simulink model "schemat_4"  (R2018a)
settings: Solver=VariableStepAuto  StartTime=0.0  StopTime=20  RelTol=1e-3
settings Model: Creator=HP  LastModifiedBy=HP

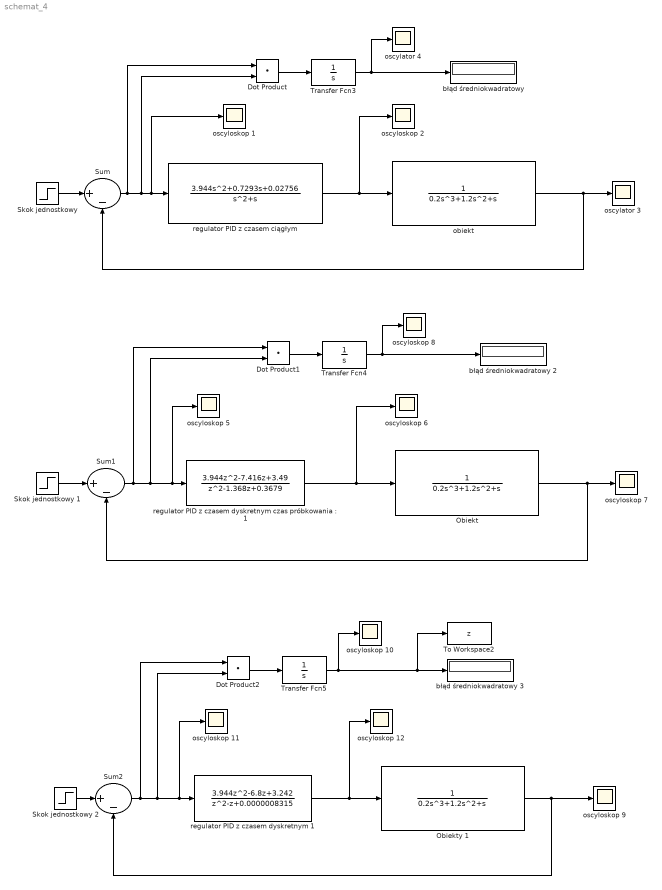
== system schemat_4 ==
  Dot Product : DotProduct  InputSameDT=on  OutDataTypeStr=Inherit: Inherit via internal rule
  Dot Product1 : DotProduct  InputSameDT=on  OutDataTypeStr=Inherit: Inherit via internal rule
  Dot Product2 : DotProduct  InputSameDT=on  OutDataTypeStr=Inherit: Inherit via internal rule
  Obiekt : TransferFcn  Denominator=[0.2 1.2 1 0]
  Obiekty 1 : TransferFcn  Denominator=[0.2 1.2 1 0]
  Skok jednostkowy : Step  SampleTime=0
  "Skok jednostkowy 1 " : Step  SampleTime=0
  Skok jednostkowy 2 : Step  SampleTime=0
  Sum : Sum  Inputs=|+-
  Sum1 : Sum  Inputs=|+-
  Sum2 : Sum  Inputs=|+-
  To Workspace2 : ToWorkspace  VariableName=z  SampleTime=-1
  Transfer Fcn3 : TransferFcn  Denominator=[1 0]
  Transfer Fcn4 : TransferFcn  Denominator=[1 0]
  Transfer Fcn5 : TransferFcn  Denominator=[1 0]
  błąd średniokwadratowy : Display
  "błąd średniokwadratowy 2 " : Display
  błąd średniokwadratowy 3 : Display
  obiekt : TransferFcn  Denominator=[0.2 1.2 1 0]
  oscylator 3 : Scope
  oscylator 4 : Scope
  oscyloskop {1..2,5..12} (10 alike) : Scope
  regulator PID z czasem ciągłym : TransferFcn  Numerator=[3.944 0.7293 0.02756]  Denominator=[1 1 0]
  "regulator PID z czasem dyskretnym czas próbkowania : 1 " : DiscreteTransferFcn  Numerator=[3.944 -7.416 3.49]  Denominator=[1 -1.368 0.3679]
  regulator PID z czasem dyskretnym 1 : DiscreteTransferFcn  Numerator=[3.944 -6.8 3.242]  Denominator=[1 -1 0.0000008315]
  wires:
  Skok jednostkowy/1 -> Sum/1
  Sum/1 -> Dot Product/1, Dot Product/2, regulator PID z czasem ciągłym/1, oscyloskop 1/1
  regulator PID z czasem ciągłym/1 -> oscyloskop 2/1, obiekt/1
  obiekt/1 -> Sum/2, oscylator 3/1
  "Skok jednostkowy 1 "/1 -> Sum1/1
  Obiekt/1 -> Sum1/2, oscyloskop 7/1
  "regulator PID z czasem dyskretnym czas próbkowania : 1 "/1 -> oscyloskop 6/1, Obiekt/1
  Dot Product/1 -> Transfer Fcn3/1
  Transfer Fcn3/1 -> oscylator 4/1, błąd średniokwadratowy/1
  Transfer Fcn4/1 -> oscyloskop 8/1, "błąd średniokwadratowy 2 "/1
  Dot Product1/1 -> Transfer Fcn4/1
  Sum1/1 -> Dot Product1/1, Dot Product1/2, "regulator PID z czasem dyskretnym czas próbkowania : 1 "/1, oscyloskop 5/1
  Sum2/1 -> Dot Product2/1, Dot Product2/2, regulator PID z czasem dyskretnym 1/1, oscyloskop 11/1
  Transfer Fcn5/1 -> błąd średniokwadratowy 3/1, To Workspace2/1, oscyloskop 10/1
  Dot Product2/1 -> Transfer Fcn5/1
  regulator PID z czasem dyskretnym 1/1 -> Obiekty 1/1, oscyloskop 12/1
  Obiekty 1/1 -> Sum2/2, oscyloskop 9/1
  Skok jednostkowy 2/1 -> Sum2/1
